simulink model "original_sim_bandpass_singleBand"  (R2024b)
settings: Solver=FixedStepDiscrete  StartTime=0.0  StopTime=(size(sm_EEG_data,1)-1)/sm.p.EEG.sr  RelTol=1e-3  EnableMultiTasking=on
values from neighbouring files (symbols this model uses):
  sm =     [reference_output.mat]
undefined symbols (not defined in the file or in its folder): fdesignblkfcn, gcbh
libraries: dspsrcs4 x1
settings Model: Creator=ronens  LastModifiedBy=hardeep
settings SolverCC: AlgebraicLoopSolver=TrustRegion
settings DataIOCC: LimitDataPoints=on  SaveFormat=Array  SignalLoggingSaveFormat=ModelDataLogs  ReturnWorkspaceOutputs=off
settings OptimizationCC: ExpressionDepthLimit=2147483647  LifeSpan=inf
settings DebuggingCC: UnderspecifiedInitializationDetection=Classic  MergeDetectMultiDrivingBlocksExec=none  SolverPrmCheckMsg=warning  ParameterPrecisionLossMsg=none  FcnCallInpInsideContextMsg=warning  UnconnectedInputMsg=warning  UnconnectedOutputMsg=warning  UnconnectedLineMsg=warning  StateNameClashWarn=warning  SFUnexpectedBacktrackingDiag=warning  SFNoUnconditionalDefaultTransitionDiag=warning  SFExecutionAtInitializationDiag=none  ArithmeticOperatorsInVariantConditions=warning
settings HardwareCC: ProdBitPerPointer=32  ProdBitPerSizeT=32  ProdBitPerPtrDiffT=32  ProdLargestAtomicFloat=None  ProdIntDivRoundTo=Undefined  ProdEndianess=Unspecified  ProdWordSize=32  ProdHWDeviceType=32-bit Generic
settings ModelReferenceCC: EnableRefExpFcnMdlSchedulingChecks=on  PropagateSignalLabelsOutOfModel=off
settings SFSimCC: SimUseLocalCustomCode=off  CustomCodeUndefinedFunction=UseInterfaceOnly
settings RTWCC: RTWUseLocalCustomCode=off  GPUComputeCapability=3.5
settings CodeAppCC: StateflowObjectComments=on
settings GRTTargetCC: TargetLangStandard=C89/C90 (ANSI)
settings ConfigComp: CovMetricSettings=dw  CovSaveCumulativeToWorkspaceVar=on  CovSaveSingleToWorkspaceVar=on  CovExternalEMLEnable=off
settings SimscapeCC: SimscapeNormalizeSystem=off
settings ConfigurationSet: Description=SimMechanics 2G

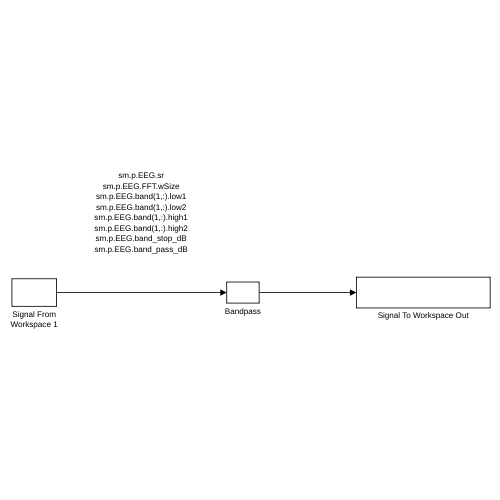
[thumbnail: Simulink's stored preview of the top-level diagram]
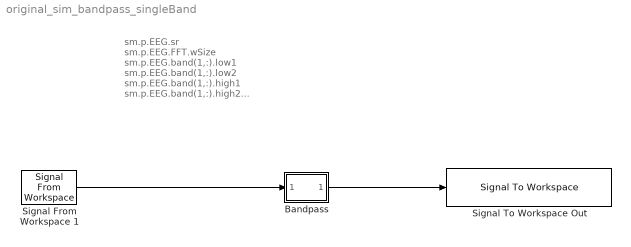
== system original_sim_bandpass_singleBand ==
  note: sm.p.EEG.sr
      | sm.p.EEG.FFT.wSize
      | sm.p.EEG.band(1,:).low1
      | sm.p.EEG.band(1,:).low2
      | sm.p.EEG.band(1,:).high1
      | sm.p.EEG.band(1,:).high2
      | sm.p.EEG.band_stop_dB
      | sm.p.EEG.band_pass_dB
  Bandpass : Subsystem
  Signal From Workspace 1 : dspsrcs4/Signal From Workspace  X=sm_EEG_data  Ts=1/sm.p.EEG.sr  nsamps=1  OutputAfterFinalValue=Setting to zero  ignoreOrWarnInputAndFrameLengths=off  OutputFrames=on
  Signal To Workspace Out : SignalToWorkspace  VariableName=Bandpass_singleBand
      settings: CopyFcn=dspblkcopystw(gcbh);
  wires:
  Signal From Workspace 1/1 -> Bandpass/1(In1)
  Bandpass/1(Out1) -> Signal To Workspace Out/1

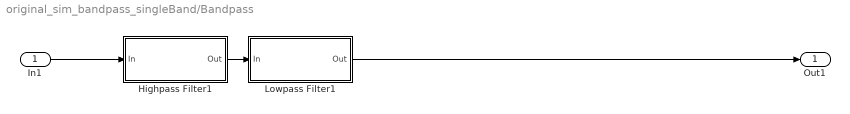
== system original_sim_bandpass_singleBand/Bandpass ==
  In1 : Inport
  Highpass Filter1 : Subsystem  DialogController=fdesignblkfcn  InitFcn=fdesignblkfcn(gcbh, {'InitFcn'});  mask(Highpass Filter){}
      mask help: Design a highpass filter
      settings: CopyFcn=fdesignblkfcn(gcbh, {'CopyFcn'});
      mask Help: helpview(mapfilelocation('dsp'), 'dsphighpassfilter');
      mask Display: disp('Highpass')
  Lowpass Filter1 : Subsystem  DialogController=fdesignblkfcn  InitFcn=fdesignblkfcn(gcbh, {'InitFcn'});  mask(Lowpass Filter){}
      mask help: Design a lowpass filter
      settings: CopyFcn=fdesignblkfcn(gcbh, {'CopyFcn'});
      mask Help: helpview(mapfilelocation('dsp'), 'dsplowpassfilter');
      mask Display: disp('Lowpass')
  Out1 : Outport
  wires:
  In1/1 -> Highpass Filter1/1(In)
  Highpass Filter1/1(Out) -> Lowpass Filter1/1(In)
  Lowpass Filter1/1(Out) -> Out1/1

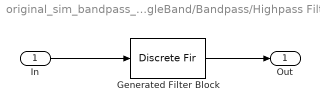
== system original_sim_bandpass_singleBand/Bandpass/Highpass Filter1 ==
  In : Inport
  Generated Filter Block : DiscreteFir  Tag=BlockMethodSubSystem  Coefficients=[0.000722557265785718603 -1.21633037762931761e-06 -0.00227651685769557398 0.00574901099488783068 -0.00822566199421323994 0.00747836565650138348 -0.00345073422616145199 -0.00119715381661103883 0.00318923327683050132 -0.00160583722907339755 -0.00128343983992251168 0.0023434544589931894 -0.000723264124794662606 -0.001486676496397476 0.00175842856999537818 3.77355172070596888e-05 -0.00164822810917868785 0.00117676987700227726 0.000697984532165207318 -0.00163773634004450892 0.00051972526049254232 0.00122077974454384342 -0.0014025819241109043 -0.000187314880191520502 0.00153726865305655333 -0.000935852393976821365 -0.000867093193554245318 0.00158519095139915108 -0.000281543808295960638 -0.00141238220799934583 0.00132875864692605979 0.000471287172315580346 -0.00171634169370658667 0.00078315197341869119 0.00119384179099407271 -0.0016944440075425519 1.87095321521616308e-05 0.00174449386626316164 -0.00131483620459773871 -0.000836584937618670664 0.00198965187441562351 -0.000608400014855880458 -0.00162035767144646202 0.00184059225918428108 0.000318659114329910989 -0.0021564825309914131 0.00127291095346570605 0.00130324663114438685 -0.00230046053831465657 0.000353257970911608702 0.0021392698525240319 -0.00196187735847893783 -0.000776322758454436163 0.0026324014762855205 -0.00115243752348438418 -0.0018930854659206988 0.00261621491256148206 3.09429732302209237e-05 -0.00276140376597828465 0.00202582046520028867 0.00138260397435366789 -0.00315537419234440111 0.000907661712747571503 0.00262741274443937731 -0.00291108648214999334 -0.000580949368571716967 0.00348416682807132149 -0.00199068389639502552 -0.00216689485593952189 0.00370313069204907105 -0.000489264263405920661 -0.003520113511275499 0.00313944077675611978 0.00135285595479369509 -0.0043055447212199064 0.00179121436596235413 0.0031875098605344712 -0.00426125886454202778 -0.000171957606371885328 0.00461174358874616094 -0.00326238408737324417 -0.00242021687655827626 0.00524543107737545505 -0.00136881507794003919 -0.0045086473464244917 0.00481557107537371708 0.00115736684097791031 -0.00595076854165700955 0.00322800761740259148 0.00387735131904113533 -0.00631692342906951896 0.000621326159234206503 0.00623071699620266449 -0.00532499934245348177 -0.00262973291160526227 0.00763619802522062102 -0.00293088698872139746 -0.00593833851628149893 0.00758963797750346076 0.000638702557931272578 -0.00860137269662461339 0.00579299561011300569 0.00486301078592909011 -0.00988960677581863547 0.0022203609450455377 0.00899980828148984682 -0.00920692303058968237 -0.00279313255610201061 0.0121357656580908958 -0.00617872133511083044 -0.00856390397537651338 0.0132954401612167834 -0.000708098413345797039 -0.0141676429692786723 0.0116521712517972734 0.00685944342551446807 -0.0183697877382836966 0.00645720208096276643 0.015892395007373987 -0.0198020578030857763 -0.00288334389871718055 0.0254500529551430696 -0.0167774816141551923 -0.0172035752547218465 0.0344607199614720208 -0.00663759405439975653 -0.0388806252884501546 0.041839406859557067 0.0180248245008368668 -0.0792155621989663605 0.0466796319450941827 0.107677763211964414 -0.296557551774083439 0.38169574423266972 -0.296557551774083439 0.107677763211964414 0.0466796319450941827 -0.0792155621989663605 0.0180248245008368668 0.041839406859557067 -0.0388806252884501546 -0.00663759405439975653 0.0344607199614720208 -0.0172035752547218465 -0.0167774816141551923 0.0254500529551430696 -0.00288334389871718055 -0.0198020578030857763 0.015892395007373987 0.00645720208096276643 -0.0183697877382836966 0.00685944342551446807 0.0116521712517972734 -0.0141676429692786723 -0.000708098413345797039 0.0132954401612167834 -0.00856390397537651338 -0.00617872133511083044 0.0121357656580908958 -0.00279313255610201061 -0.00920692303058968237 0.00899980828148984682 0.0022203609450455377 -0.00988960677581863547 0.00486301078592909011 0.00579299561011300569 -0.00860137269662461339 0.000638702557931272578 0.00758963797750346076 -0.00593833851628149893 -0.00293088698872139746 ...(+2264 chars)]  InputProcessing=Columns as channels (frame based)
  Out : Outport
  wires:
  Generated Filter Block/1 -> Out/1
  In/1 -> Generated Filter Block/1

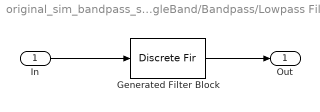
== system original_sim_bandpass_singleBand/Bandpass/Lowpass Filter1 ==
  In : Inport
  Generated Filter Block : DiscreteFir  Tag=BlockMethodSubSystem  Coefficients=[0.0051163137049697301 0.00664912466311140885 -0.00659888443703180502 -0.0173299101318000574 -0.00766144205918836436 0.00127351369274435709 -0.00438460058803490267 -0.00437297847863413712 0.00204860812540660778 -0.000937682552100423117 -0.00291988035593412605 0.00183688406261209433 0.000115289284565135968 -0.00231511602211972346 0.00154600094079728845 0.00048036491188303761 -0.00204974834039397397 0.0013318262230916306 0.000639092394607129809 -0.00193998700308905961 0.00119316825416292301 0.000744372466337165479 -0.00191226160140160425 0.00110085995628469817 0.000841082862656065446 -0.00193285662979430779 0.00103811847304926901 0.000948473845809220863 -0.00198541724549032702 0.000985938833038452461 0.00106431450956237495 -0.00206304906487311682 0.0009435443776796465 0.00120287977846118854 -0.00215864701788916419 0.000896626876166414896 0.00135879593704738943 -0.00226758983689367933 0.000839785842861324149 0.00153194845875738971 -0.00238498991968584192 0.000774976758590589896 0.00172307599426980008 -0.00250936246738788817 0.000698158762509018972 0.00193422011561939573 -0.00263840418239885948 0.00060769990345491793 0.00216399401554065365 -0.00277462948071386696 0.000497626733984523153 0.00241262212668373957 -0.00291136175450415523 0.000373215665265861263 0.00268502962182890371 -0.00305404110891653591 0.000222167918534272083 0.00297939873987107832 -0.00319672223460916319 4.75454663399570743e-05 0.00329988215267934884 -0.00333472977538297943 -0.000150620422748928682 0.00364572614841406593 -0.00347658358296222764 -0.00038392599781110709 0.00402321410232760798 -0.00360536060649413416 -0.000643704517505494446 0.00442792905174549303 -0.0037392016131287337 -0.000943336184010563645 0.00487233158038579729 -0.00386183677786745665 -0.00128151439176165793 0.00535310895108082573 -0.00398561506899764665 -0.00166961543496784359 0.00588156383981101177 -0.00410534241095077135 -0.00211468989786104018 0.00646507399263940557 -0.00422126939152915343 -0.00262817946235640492 0.00711315061095691217 -0.00433649335119125866 -0.0032265286116043017 0.00784782451597193335 -0.00443353583629501908 -0.00392040976887024235 0.00867120126025416708 -0.00454354693377290782 -0.00474243757334357873 0.00965203862766068552 -0.00461028873164573763 -0.0057242752838001891 0.0107622817795137039 -0.00470685848565745735 -0.00691537946174597233 0.0121365692683771016 -0.00477025645420156748 -0.0084049912432620031 0.0138130580358613066 -0.00483799300835138606 -0.0103213649274392534 0.015952647848410207 -0.00490836362928324336 -0.0128667919200813399 0.0188626214774604804 -0.00495738056511318189 -0.016469622949095878 0.0230244581685182387 -0.00499333919808033887 -0.0219844984442896206 0.0295530095820308418 -0.00502076461390900397 -0.0315257991397836293 0.0415271050460503249 -0.00504418809697514559 -0.0523397053931333803 0.0712298721652367822 -0.00506296473777317207 -0.135190576730842282 0.278143682298504613 0.661594525215955853 0.278143682298504613 -0.135190576730842282 -0.00506296473777317207 0.0712298721652367822 -0.0523397053931333803 -0.00504418809697514559 0.0415271050460503249 -0.0315257991397836293 -0.00502076461390900397 0.0295530095820308418 -0.0219844984442896206 -0.00499333919808033887 0.0230244581685182387 -0.016469622949095878 -0.00495738056511318189 0.0188626214774604804 -0.0128667919200813399 -0.00490836362928324336 0.015952647848410207 -0.0103213649274392534 -0.00483799300835138606 0.0138130580358613066 -0.0084049912432620031 -0.00477025645420156748 0.0121365692683771016 -0.00691537946174597233 -0.00470685848565745735 0.0107622817795137039 -0.0057242752838001891 -0.00461028873164573763 0.00965203862766068552 -0.00474243757334357873 -0.00454354693377290782 0.00867120126025416708 -0.00392040976887024235 -0.00443353583629501908 0.00784782451597193335 -0.0032265286116043017 -0.00433649335119125866 0.00711315061095691217 -0.00262817946235640492 -0.00422126939152915343 0.00646507399263940557 -0.00211468989786104018 -0.00410534241095077135 0.00588156383981101177 ...(+1842 chars)]  InputProcessing=Columns as channels (frame based)
  Out : Outport
  wires:
  In/1 -> Generated Filter Block/1
  Generated Filter Block/1 -> Out/1
